simulink model "Prob3ISTR"  (R2019b)
settings: Solver=VariableStepAuto  StartTime=0.0  StopTime=200  RelTol=1e-3
values from neighbouring files (symbols this model uses):
  am1 = -1.3205    [discrete1.m]    (also in discrete2.m; dstr_demo.m; istr.m)
  am2 = 0.4966    [discrete1.m]    (also in discrete2.m; dstr_demo.m; istr.m)
  lambda = 0.95    [discrete1.m]    (also in dstr_demo.m = 0.98; istr.m = 0.1)
  P0 = 100*eye(4)    [discrete1.m]    (also in istr.m = diag([10000,10000,10000,10000]))
  teta0 = [-1.5 0.5 2 2]    [discrete1.m]    (also in istr.m = [-1.5 0.5 -2 -2])
undefined symbols (not defined in the file or in its folder): den, num
settings Model: Creator=nadimkhairallah  LastModifiedBy=ramzih15
settings DataIOCC: ReturnWorkspaceOutputs=off
settings DebuggingCC: ArithmeticOperatorsInVariantConditions=warning
settings SFSimCC: SimUseLocalCustomCode=off  CustomCodeUndefinedFunction=UseInterfaceOnly
settings RTWCC: RTWUseLocalCustomCode=off

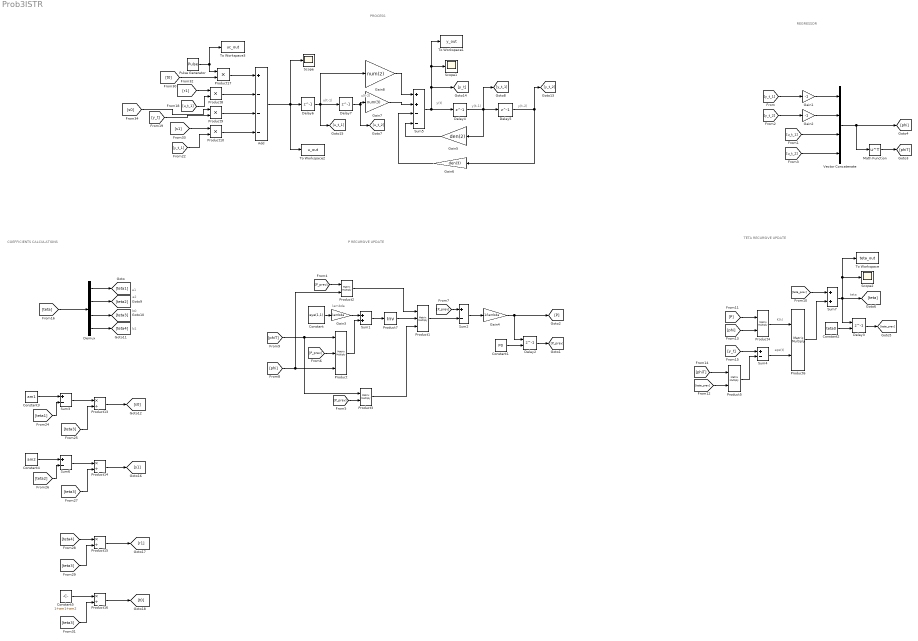
== system Prob3ISTR ==
  note: COEFFICIENTS CALCULATIONS
  note: b1
  note: b0
  note: a2
  note: a1
  note: REGRESSOR
  note: eps(t)
  note: teta
  note: TETA RECURSIVE UPDATE
  note: P RECURSIVE UPDATE
  note: y(t-1)
  note: y(t)
  note: K(t)
  note: lambda
  note: u(t-2)
  note: u(t-1)
  note: y(t-2)
  note: PROCESS
  Add : Sum  Inputs=+---
  Constant : Constant  Value=eye(1,1)
  Constant1 : Constant  Value=P0
  Constant2 : Constant  Value=teta0
  Constant3 : Constant  Value=am1
  Constant4 : Constant  Value=am2
  Constant5 : Constant  Value=1+am1+am2
  Delay2 : Delay  DelayLength=1  InitialConditionSource=Input port  InitialCondition=0
      settings: InputPortMap=u0,p4
  Delay3 : Delay  DelayLength=1  InitialConditionSource=Input port  InitialCondition=0
      settings: InputPortMap=u0,p4
  Delay{4..7} (4 alike) : Delay  DelayLength=1  InitialCondition=0
  Demux : Demux
  Gain1 : Gain  Gain=-1
  Gain2 : Gain  Gain=-1
  Gain3 : Gain  Gain=lambda
  Gain4 : Gain  Gain=1/lambda
  Gain5 : Gain  Gain=den(2)
  Gain6 : Gain  Gain=den(3)
  Gain7 : Gain  Gain=num(3)
  Gain8 : Gain  Gain=num(2)
  Math Function : Math  Operator=transpose  SaturateOnIntegerOverflow=on
  Product : Product  Inputs=3  Multiplication=Matrix(*)
  Product1 : Product  Inputs=3  Multiplication=Matrix(*)
  Product{8..10,17} (4 alike) : Product
  Product{13..16} (4 alike) : Product  Inputs=*/
  Product{2..6} (5 alike) : Product  Multiplication=Matrix(*)
  Product7 : Product  Inputs=/  Multiplication=Matrix(*)
  Pulse Generator : DiscretePulseGenerator  Period=40  PulseWidth=20
  Scope : Scope
  Scope1 : Scope
  Scope2 : Scope
  Sum1 : Sum
  Sum{2..4,6} (4 alike) : Sum  Inputs=+-
  Sum5 : Sum  Inputs=++--
  Sum7 : Sum
  To Workspace : ToWorkspace  VariableName=teta_out  SampleTime=-1
  To Workspace1 : ToWorkspace  VariableName=y_out  SampleTime=-1
  To Workspace2 : ToWorkspace  VariableName=u_out  SampleTime=-1
  To Workspace3 : ToWorkspace  VariableName=uc_out  SampleTime=-1
  Vector Concatenate : Concatenate  NumInputs=4
  wires:
  Vector Concatenate/1 -> Math Function/1, [phi]
  Gain5/1 -> Sum5/4
  Product6/1 -> Sum7/2
  Product2/1 -> Product1/1
  Add/1 -> Scope/1, To Workspace2/1, Delay6/1
  Demux/2 -> [teta2]
  [phiT] -> Product5/1
  Product9/1 -> Add/3
  Constant1/1 -> Delay2/2
  [phi] -> Product4/2
  Math Function/1 -> [phiT]
  [P_prev] -> Product/2
  Constant2/1 -> Delay3/2
  Sum4/1 -> Product6/2
  Gain6/1 -> Sum5/3
  Delay3/1 -> [teta_prev]
  [teta_prev] -> Sum7/1
  Sum1/1 -> Product7/1
  Sum7/1 -> To Workspace/1, Scope2/1, [teta], Delay3/1
  [phiT] -> Product3/1, Product/1
  Product5/1 -> Sum4/2
  Product10/1 -> Add/4
  Demux/1 -> [teta1]
  Gain4/1 -> [P], Delay2/1
  [y_t] -> Sum4/1
  Gain8/1 -> Sum5/1
  Product7/1 -> Product1/2
  Constant/1 -> Gain3/1
  [P_prev] -> Product2/1
  [teta_prev] -> Product5/2
  Product17/1 -> Add/1
  [phi] -> Product2/2, Product/3
  Product4/1 -> Product6/1
  Delay7/1 -> [u_t_2], Gain7/1
  Product/1 -> Sum1/2
  [P_prev] -> Product3/2
  Gain3/1 -> Sum1/1
  Product1/1 -> Sum2/2
  Delay6/1 -> Delay7/1, [u_t_1], Gain8/1
  Gain7/1 -> Sum5/2
  Delay4/1 -> [y_t_1], Gain5/1, Delay5/1
  [P_prev] -> Sum2/1
  Delay5/1 -> [y_t_2], Gain6/1
  Sum2/1 -> Gain4/1
  Product3/1 -> Product1/3
  Sum5/1 -> [y_t], To Workspace1/1, Scope1/1, Delay4/1
  Demux/3 -> [teta3]
  [y_t_1] -> Product10/2
  Delay2/1 -> [P_prev]
  [u_t_1] -> Product8/2
  [s0] -> Product9/1
  [r1] -> Product8/1
  [y_t] -> Product9/2
  Product8/1 -> Add/2
  [P] -> Product4/1
  [teta] -> Demux/1
  Pulse Generator/1 -> To Workspace3/1, Product17/1
  [s1] -> Product10/1
  [y_t_1] -> Gain1/1
  Gain1/1 -> Vector Concatenate/1
  [y_t_2] -> Gain2/1
  Gain2/1 -> Vector Concatenate/2
  [u_t_2] -> Vector Concatenate/4
  [u_t_1] -> Vector Concatenate/3
  Constant3/1 -> Sum3/1
  [teta1] -> Sum3/2
  Sum3/1 -> Product13/1
  [teta3] -> Product13/2
  Demux/4 -> [teta4]
  Product13/1 -> [s0]
  Product14/1 -> [s1]
  [teta3] -> Product14/2
  Sum6/1 -> Product14/1
  [teta2] -> Sum6/2
  Constant4/1 -> Sum6/1
  Product15/1 -> [r1]
  [teta4] -> Product15/1
  [teta3] -> Product15/2
  [teta3] -> Product16/2
  Product16/1 -> [t0]
  Constant5/1 -> Product16/1
  [t0] -> Product17/2
